simulink model "LQI"  (R2021a)
settings: Solver=VariableStepAuto  StartTime=0.0  StopTime=500  RelTol=1e-3
values from neighbouring files (symbols this model uses):
  A = [-0.0299243213669892 0.0256028069981396 ... (first row only)    [m3007.m]    (also in process_parameters.m = [-1/Tv, 0, 0; real_data_2.m = [-1/Tv, 0, 0; rls_algorithm.m = [-1/Tv, 0, 0)
  A1 = 450    [process_parameters.m]    (also in real_data_2.m; rls_algorithm.m)
  B = [0.00171378115848002; 0]    [m3007.m]    (also in process_parameters.m = [Kv/Tv; 0; 0]; real_data_2.m = [Kv/Tv; 0; 0]; rls_algorithm.m = [Kv/Tv; 0; 0])
  C = [0, 1]    [m3007.m]    (also in process_parameters.m = [0, 0, 1]; real_data_2.m = [0, 0, 1]; rls_algorithm.m = [0, 0, 1])
  g = 981    [process_parameters.m]    (also in real_data_2.m; rls_algorithm.m)
  h10 = data.WaterLevelTank1(start_index)    [m3007.m]    (also in process_parameters.m = 4.69; real_data_2.m = 4.69; rls_algorithm.m = 4.69)
  h20 = data.WaterLevelTank2(start_index)    [m3007.m]    (also in process_parameters.m = 3.39; real_data_2.m = 3.39; rls_algorithm.m = 3.39)
  K12A = K3*A1/sqrt(2*g)    [process_parameters.m]    (also in real_data_2.m; rls_algorithm.m)
  K12B = K2*A1/sqrt(2*g)    [process_parameters.m]    (also in real_data_2.m; rls_algorithm.m)
  K1d = K4*A1/sqrt(2*g)    [process_parameters.m]    (also in real_data_2.m; rls_algorithm.m)
  K2d = K4*A1/sqrt(2*g)    [process_parameters.m]    (also in real_data_2.m; rls_algorithm.m)
  Ki = K1*A1/sqrt(2*g)    [process_parameters.m]    (also in real_data_2.m; rls_algorithm.m)
  Kii = Kpoj(:, 4)    [LQI_controller.m]
  Kv = 3.0519 + 0.3    (= 3.3519)    [process_parameters.m]    (also in real_data_2.m = 3.2519; rls_algorithm.m = 3.2519)
  Kx = Kpoj(:, 1:3)    [LQI_controller.m]
  qu0 = data.InletFlow(start_index)*(1000/60)    [m3007.m]    (also in process_parameters.m = 93; real_data_2.m = 82; rls_algorithm.m = 82)
  Tv = 1.74    [process_parameters.m]    (also in real_data_2.m; rls_algorithm.m)
  xv0 = 25    [process_parameters.m]    (also in real_data_2.m; rls_algorithm.m)
settings Model: Creator=matij  LastModifiedBy=matij

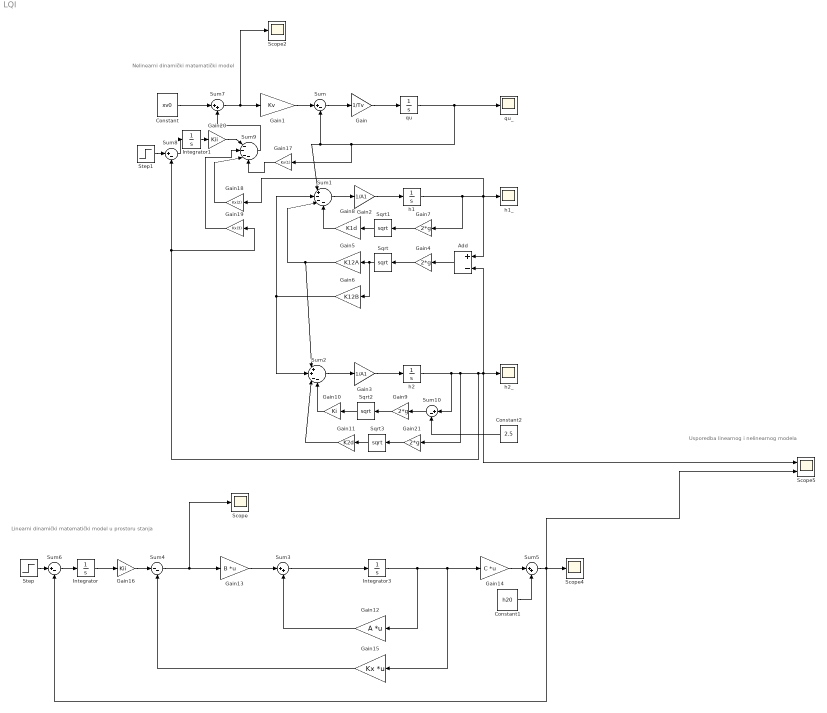
== system LQI ==
  note: Nelinearni dinamički matematički model
  note: Linearni dinamički matematički model u prostoru stanja
  note: Usporedba linearnog i nelinearnog modela
  Add : Sum  Inputs=+-
  Constant : Constant  Value=xv0
  Constant1 : Constant  Value=h20
  Constant2 : Constant  Value=2.5
  Gain : Gain  Gain=1/Tv
  Gain1 : Gain  Gain=Kv
  Gain10 : Gain  Gain=Ki
  Gain11 : Gain  Gain=K2d
  Gain12 : Gain  Gain=A  Multiplication=Matrix(K*u)
  Gain13 : Gain  Gain=B  Multiplication=Matrix(K*u)
  Gain14 : Gain  Gain=C  Multiplication=Matrix(K*u)
  Gain15 : Gain  Gain=Kx  Multiplication=Matrix(K*u)
  Gain16 : Gain  Gain=Kii
  Gain17 : Gain  Gain=Kx(1)
  Gain18 : Gain  Gain=Kx(2)
  Gain19 : Gain  Gain=Kx(3)
  Gain2 : Gain  Gain=1/A1
  Gain20 : Gain  Gain=Kii
  Gain{4,7,9,21} (4 alike) : Gain  Gain=2*g
  Gain3 : Gain  Gain=1/A1
  Gain5 : Gain  Gain=K12A
  Gain6 : Gain  Gain=K12B
  Gain8 : Gain  Gain=K1d
  Integrator : Integrator
  Integrator1 : Integrator
  Integrator3 : Integrator
  Scope : Scope
  Scope2 : Scope
  Scope4 : Scope
  Scope5 : Scope  NumInputPorts=2
  Sqrt{,1..3} (4 alike) : Sqrt  SaturateOnIntegerOverflow=on
  Step : Step  Before=h20  After=h20+20  SampleTime=0
  Step1 : Step  Time=0  Before=h20  After=h20+20  SampleTime=0
  Sum{,6,8,10} (4 alike) : Sum  Inputs=|+-
  Sum1 : Sum  Inputs=|+---
  Sum2 : Sum  Inputs=|++--
  Sum3 : Sum  Inputs=|++
  Sum4 : Sum  Inputs=|--
  Sum5 : Sum  Inputs=|++
  Sum7 : Sum  Inputs=|++
  Sum9 : Sum  Inputs=|----
  h1 : Integrator  InitialCondition=h10
  h1_ : Scope
  h2 : Integrator  InitialCondition=h20
  h2_ : Scope
  qu : Integrator  InitialCondition=qu0
  qu_ : Scope
  wires:
  Add/1 -> Gain4/1
  Gain10/1 -> Sum2/4
  Sqrt/1 -> Gain6/1, Gain5/1
  Gain12/1 -> Sum3/2
  Sum1/1 -> Gain2/1
  Integrator3/1 -> Gain15/1, Gain14/1, Gain12/1
  Sum5/1 -> Scope4/1, Sum6/2, Scope5/2
  Gain13/1 -> Sum3/1
  Gain2/1 -> h1/1
  Gain6/1 -> Sum2/2, Sum1/2
  Gain5/1 -> Sum1/3, Sum2/1
  Gain9/1 -> Sqrt2/1
  Sqrt2/1 -> Gain10/1
  h2/1 -> Sum10/1, Gain21/1, Gain19/1, Sum8/2, Scope5/1, Add/2, h2_/1
  Sqrt1/1 -> Gain8/1
  Gain4/1 -> Sqrt/1
  Sum3/1 -> Integrator3/1
  Constant1/1 -> Sum5/2
  Gain8/1 -> Sum1/4
  Sum/1 -> Gain/1
  Sum4/1 -> Scope/1, Gain13/1
  Sum2/1 -> Gain3/1
  qu/1 -> Gain17/1, Sum1/1, Sum/2, qu_/1
  Gain11/1 -> Sum2/3
  h1/1 -> Gain18/1, h1_/1, Add/1, Gain7/1
  Gain1/1 -> Sum/1
  Gain/1 -> qu/1
  Gain7/1 -> Sqrt1/1
  Gain14/1 -> Sum5/1
  Gain3/1 -> h2/1
  Gain15/1 -> Sum4/2
  Gain16/1 -> Sum4/1
  Integrator/1 -> Gain16/1
  Sum6/1 -> Integrator/1
  Constant/1 -> Sum7/1
  Sum7/1 -> Scope2/1, Gain1/1
  Step/1 -> Sum6/1
  Step1/1 -> Sum8/1
  Sum9/1 -> Sum7/2
  Gain17/1 -> Sum9/4
  Gain18/1 -> Sum9/3
  Gain19/1 -> Sum9/2
  Gain20/1 -> Sum9/1
  Integrator1/1 -> Gain20/1
  Sum8/1 -> Integrator1/1
  Sqrt3/1 -> Gain11/1
  Gain21/1 -> Sqrt3/1
  Sum10/1 -> Gain9/1
  Constant2/1 -> Sum10/2
